simulink model "rtwdemo_ssreuse"  (Simulink 7.6)
settings: Solver=FixedStepDiscrete  StartTime=0.0  StopTime=10.0  RelTol=1e-3  SampleTimeConstraint=STIndependent
PreLoadFcn:
  | rtwdemo_ssreuse_data
undefined symbols (not defined in the file or in its folder): T1Break, T1Data, T2Break, T2Data
libraries: rtwdemowidgets x2
Description:
  | Reusing Functions in Generated Code
settings Model: Creator=The MathWorks Inc.  ExtModeAutoUpdateStatusClock=off
settings DataIOCC: SaveOutput=off  SaveTime=off  SignalLoggingName=sigsOut
settings OptimizationCC: InlineParams=on  InlineInvariantSignals=on  StateBitsets=on  DataBitsets=on  UseTempVars=on  EfficientFloat2IntCast=on  EfficientMapNaN2IntZero=off
settings DebuggingCC: CheckExecutionContextPreStartOutputMsg=on  CheckExecutionContextRuntimeOutputMsg=on  SolverPrmCheckMsg=none  StrictBusMsg=ErrorOnBusTreatedAsVector
settings HardwareCC: ProdIntDivRoundTo=Zero  ProdEndianess=LittleEndian  ProdHWDeviceType=Generic->32-bit Embedded Processor  TargetHWDeviceType=Generic->32-bit Embedded Processor
settings RTWCC: TLCOptions=-p0 -aWarnNonSaturatedBlocks=0  GenerateReport=on  RTWVerbose=off  ProcessScript=grt_make_rtw_hook  LaunchReport=on
settings CodeAppCC: ForceParamTrailComments=on
settings GRTTargetCC: TargetFcnLib=ansi_tfl_tmw.mat

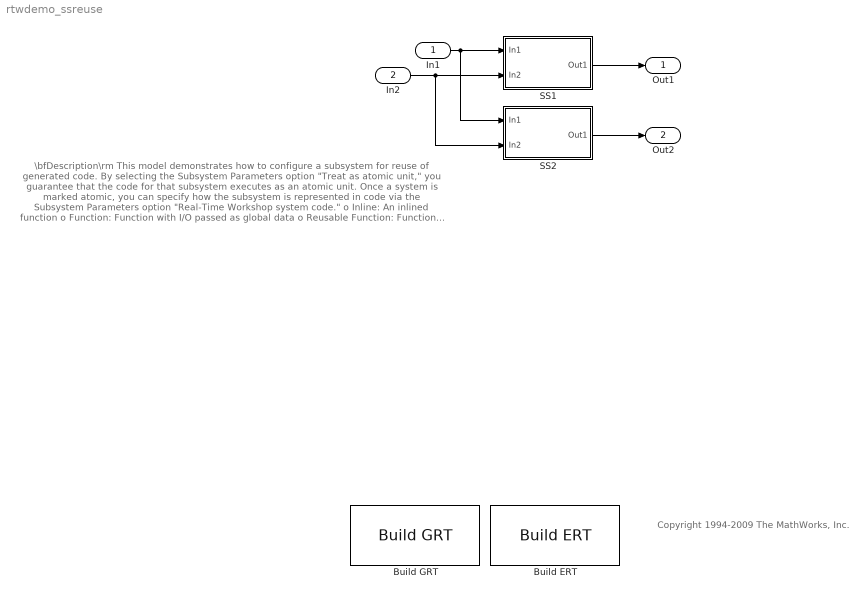
== system rtwdemo_ssreuse ==
  note: \bfDescription\rm
      | This model demonstrates how to configure a subsystem for reuse of generated code.  By selecting the
      | Subsystem Parameters option "Treat as atomic unit," you guarantee that the code for that subsystem
      | executes as an atomic unit.  Once a system is marked atomic, you can specify how the subsystem is
      | represented in code via the Subsystem Parameters option "Real-Time Workshop system code."
      |
      | o  Inline:  An inlined function
      | o  Function:  Function with I/O passed as global data
      | o  Reusable Function:  Function with I/O passed as function arguments
      | o  Auto:  Let Real-Time Workshop optimize based on context
      |
      | The last two options permit Simulink to reuse the subsystem in the generated code.  The function name
      | is controlled with the "Real-Time Workshop function name" option.  Here, SS2 is simply a copy of SS1,
      | which is configured as a "Reusable Function" with function name "myfun".  Notice that the system is a
      | parameterized masked subsystem. Parameters of a mask become arguments to the function.  This
      | example uses parameters: T1Break, T1Data, T2Break, and T2Data.
      |
      | \bfInstructions\rm
      | To see the subsystem parameters, right-click the subsystem block and select "SubSystem Parameters."
      | To see the content of the masked subsystem, right-click the subsystem block and select "Look Under Mask."
  note: Copyright 1994-2009 The MathWorks, Inc.
  In1 : Inport  OutDataTypeStr=double  PortDimensions=1
  In2 : Inport  Port=2  OutDataTypeStr=double  PortDimensions=1
  Build ERT : rtwdemowidgets/Build ERT  SystemSampleTime=-1  attrib_overrides={}
  Build GRT : rtwdemowidgets/Build GRT  SystemSampleTime=-1  attrib_overrides={}
  SS1 : Subsystem  TreatAsAtomicUnit=on  RTWFcnName=myfun  RTWFileName=myfile  mask(SSDemo){x=T1Break, y=T1Data}
      mask prompts: x "Break points (X data):"; y "Output values (Y data):"
      mask help: Example to demonstrate code reuse. This example has two parameters for a lookup table.
      settings: RTWFcnNameOpts=User specified
  SS2 : Subsystem  TreatAsAtomicUnit=on  RTWFcnName=myfun  RTWFileName=myfile  mask(SSDemo){x=T2Break, y=T2Data}
      mask prompts: x "Break points (X data):"; y "Output values (Y data):"
      mask help: Example to demonstrate code reuse. This example has two parameters for a lookup table.
      settings: RTWFcnNameOpts=User specified
  Out1 : Outport
  Out2 : Outport  Port=2
  wires:
  SS1/1(Out1) -> Out1/1
  In2/1 -> SS1/2(In2), SS2/2(In2)
  In1/1 -> SS1/1(In1), SS2/1(In1)
  SS2/1(Out1) -> Out2/1

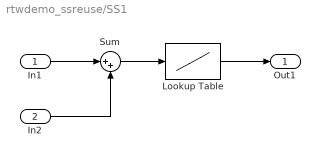
== system rtwdemo_ssreuse/SS1 ==
  In1 : Inport
  In2 : Inport  Port=2
  Lookup Table : Lookup  InputValues=x  Table=y
  Sum : Sum  Inputs=|++
  Out1 : Outport
  wires:
  In1/1 -> Sum/1
  Lookup Table/1 -> Out1/1
  In2/1 -> Sum/2
  Sum/1 -> Lookup Table/1

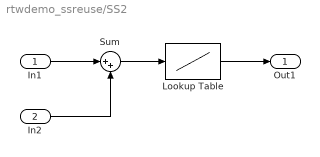
== system rtwdemo_ssreuse/SS2 ==
  In1 : Inport
  In2 : Inport  Port=2
  Lookup Table : Lookup  InputValues=x  Table=y
  Sum : Sum  Inputs=|++
  Out1 : Outport
  wires:
  Sum/1 -> Lookup Table/1
  In2/1 -> Sum/2
  Lookup Table/1 -> Out1/1
  In1/1 -> Sum/1
